simulink model "modular_NL_Modell_2020b"  (R2020b)
settings: Solver=VariableStepAuto  StartTime=0.0  StopTime=15  RelTol=1e-3
undefined symbols (not defined in the file): L_0, r1, r2, T1, T2, ue1, ue2, x_0
libraries: simulink x2, simulink_extras x2
settings Model: Creator=Patrick  LastModifiedBy=Fritz
settings DataIOCC: ReturnWorkspaceOutputs=off
settings DebuggingCC: ArithmeticOperatorsInVariantConditions=warning
settings SFSimCC: SimUseLocalCustomCode=off  CustomCodeUndefinedFunction=UseInterfaceOnly
settings RTWCC: RTWUseLocalCustomCode=off
settings CodeAppCC: StateflowObjectComments=on

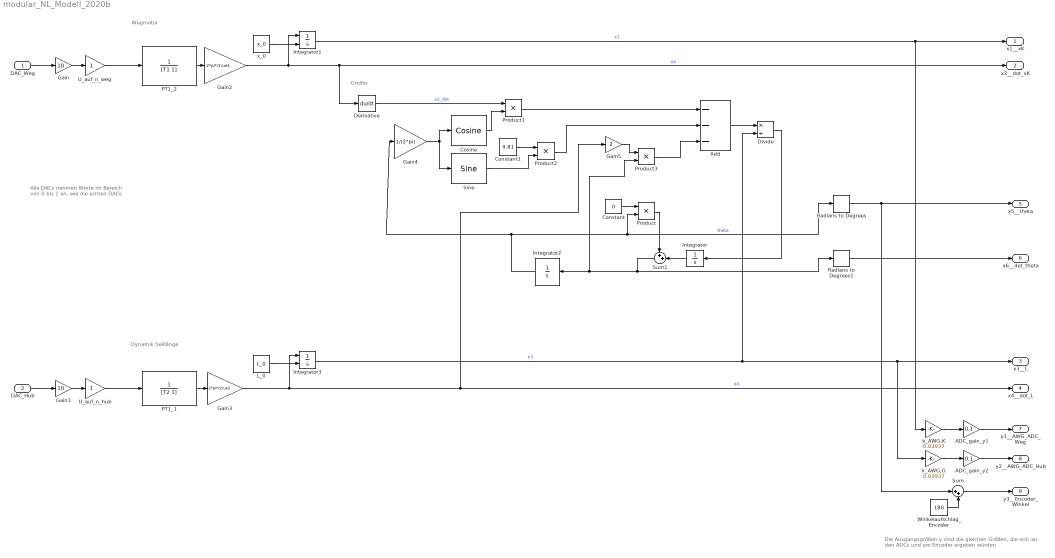
== system modular_NL_Modell_2020b ==
  note: Greifer
  note: Wegmotor
  note: Dynamik Seillänge
  note: Die Ausgangsgrößen y sind die gleichen Größen,
      | die sich an den ADCs und am Encoder ergeben würden
  note: Alle DACs nehmen Werte im Bereich
      | von 0 bis 1 an, wie die echten DACs
  DAC_Weg : Inport
  DAC_Hub : Inport  Port=2
  ADC_gain_y1 : Gain  Gain=0.1
  ADC_gain_y2 : Gain  Gain=0.1
  Add : Sum  Inputs=---
  Constant : Constant  Value=0
  Constant1 : Constant  Value=9.81
  Cosine : simulink/Lookup Tables/Cosine  Formula=cos(2*pi*u)  NumDataPoints=(2^5)+1  OutputWordLength=16  InternalRulePriority=Speed
      settings: SourceProductBaseCode=SL
  Derivative : Derivative
  Divide : Product  Inputs=*/
  Gain : Gain  Gain=10
  Gain1 : Gain  Gain=10
  Gain2 : Gain  Gain=2*pi*r1/ue1
  Gain3 : Gain  Gain=2*pi*r2/ue2
  Gain4 : Gain  Gain=1/(2*pi)
  Gain5 : Gain  Gain=2
  Integrator : Integrator
  Integrator1 : Integrator  InitialConditionSource=external
  Integrator2 : Integrator
  Integrator3 : Integrator  InitialConditionSource=external
  L_0 : Constant  Value=L_0
  PT1_1 : TransferFcn  Denominator=[T2 1]
  PT1_2 : TransferFcn  Denominator=[T1 1]
  Product{,1..3} (4 alike) : Product
  Radians to Degrees : simulink_extras/Transformations/Radians to Degrees
  Radians to Degrees1 : simulink_extras/Transformations/Radians to Degrees
  Sine : simulink/Lookup Tables/Sine  Formula=sin(2*pi*u)  NumDataPoints=(2^5)+1  OutputWordLength=16  InternalRulePriority=Speed
  Sum : Sum  Inputs=|++
  Sum1 : Sum  Inputs=++|
  U_auf_n_hub : Gain
  U_auf_n_weg : Gain
  Winkelaufschlag_Encoder : Constant  Value=180
  k_AWG,G : Gain  Gain=0.03937
  k_AWG,K : Gain  Gain=0.03937
  x_0 : Constant  Value=x_0
  x1__xK : Outport  SignalName=x1__xK
  x2__dot_xK : Outport  Port=2  SignalName=x2__dot_xK
  x3__L : Outport  Port=3  SignalName=x3__L
  x4__dot_L : Outport  Port=4  SignalName=x4__dot_L
  x5__theta : Outport  Port=5  SignalName=x5__theta
  x6__dot_theta : Outport  Port=6  SignalName=x6__dot_theta
  y1__AWG_ADC_Weg : Outport  Port=7  SignalName=y1__AWG_ADC_Weg
  y2__AWG_ADC_Hub : Outport  Port=8  SignalName=y2__AWG_ADC_Hub
  y3__Encoder_Winkel : Outport  Port=9  SignalName=y3__Encoder_Winkel
  wires:
  Integrator2/1 -> Gain4/1, Product/2, Radians to Degrees/1  "theta"
  Sum1/1 -> Radians to Degrees1/1, Integrator2/1, Product3/2
  Radians to Degrees1/1 -> x6__dot_theta/1
  Integrator1/1 -> k_AWG,K/1, x1__xK/1  "x1"
  Radians to Degrees/1 -> x5__theta/1, Sum/1
  k_AWG,K/1 -> ADC_gain_y1/1
  k_AWG,G/1 -> ADC_gain_y2/1
  Winkelaufschlag_Encoder/1 -> Sum/2
  Sum/1 -> y3__Encoder_Winkel/1
  ADC_gain_y2/1 -> y2__AWG_ADC_Hub/1
  ADC_gain_y1/1 -> y1__AWG_ADC_Weg/1
  DAC_Weg/1 -> Gain/1
  Gain/1 -> U_auf_n_weg/1
  DAC_Hub/1 -> Gain1/1
  Gain1/1 -> U_auf_n_hub/1
  L_0/1 -> Integrator3/2
  PT1_1/1 -> Gain3/1
  U_auf_n_hub/1 -> PT1_1/1
  PT1_2/1 -> Gain2/1
  U_auf_n_weg/1 -> PT1_2/1
  x_0/1 -> Integrator1/2
  Product/1 -> Sum1/1
  Integrator/1 -> Sum1/2
  Gain2/1 -> x2__dot_xK/1, Derivative/1, Integrator1/1  "x2"
  Constant/1 -> Product/1
  Gain3/1 -> Integrator3/1, x4__dot_L/1, Gain5/1  "x4"
  Integrator3/1 -> Divide/2, k_AWG,G/1, x3__L/1  "x3"
  Derivative/1 -> Product1/1  "x2_dot"
  Gain4/1 -> Sine/1, Cosine/1
  Cosine/1 -> Product1/2
  Product1/1 -> Add/1
  Constant1/1 -> Product2/1
  Sine/1 -> Product2/2
  Product2/1 -> Add/2
  Gain5/1 -> Product3/1
  Product3/1 -> Add/3
  Add/1 -> Divide/1
  Divide/1 -> Integrator/1
